simulink model "MaglevOld"  (R2015a)
settings: Solver=ode45  StartTime=0.0  StopTime=10.0  RelTol=1e-3
InitFcn:
  | m = 0.025; % kg
  | g = 9.8; % m/s2
  | L = 0.02; % H
  | R = 4.2; % ohms
  | k = 2.35; % N2/A2
undefined symbols (not defined in the file or in its folder): magnitude
settings Model: Creator=Logan  LastModifiedBy=Logan

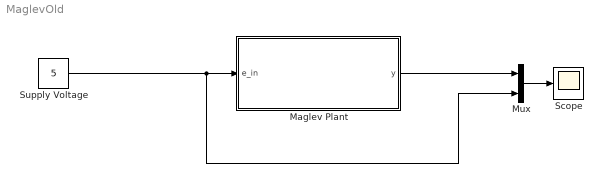
== system MaglevOld ==
  Maglev Plant : Subsystem
  Mux : Mux  Inputs=2
  Scope : Scope
  Supply Voltage : Constant  Value=5
  wires:
  Supply Voltage/1 -> Mux/2, Maglev Plant/1(e_in)
  Maglev Plant/1(y) -> Mux/1
  Mux/1 -> Scope/1

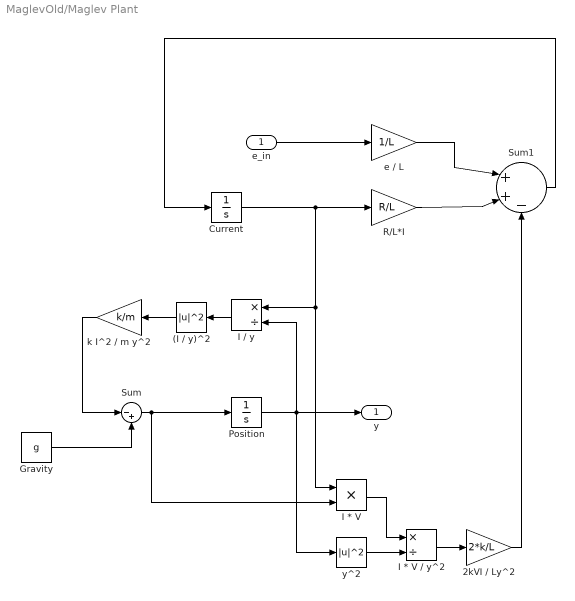
== system MaglevOld/Maglev Plant ==
  e_in : Inport
  (I / y)^2 : Math  Operator=magnitude^2  SaturateOnIntegerOverflow=on
  2kVI / Ly^2 : Gain  Gain=2*k/L
  Current : Integrator  InitialCondition=3.2
  Gravity : Constant  Value=g
  I * V : Product
  I * V / y^2 : Product  Inputs=*/
  I / y : Product  Inputs=*/
  Position : Integrator  InitialCondition=0.01  LimitOutput=on  LowerSaturationLimit=0
  R/L*I : Gain  Gain=R/L
  Sum : Sum  Inputs=|-+
  Sum1 : Sum  Inputs=|++-
  e / L : Gain  Gain=1/L
  k I^2 / m y^2 : Gain  Gain=k/m
  y^2 : Math  Operator=magnitude^2  SaturateOnIntegerOverflow=on
  y : Outport
  wires:
  2kVI / Ly^2/1 -> Sum1/3
  e_in/1 -> e / L/1
  (I / y)^2/1 -> k I^2 / m y^2/1
  e / L/1 -> Sum1/1
  k I^2 / m y^2/1 -> Sum/1
  Sum/1 -> I * V/2, Position/1
  Position/1 -> y^2/1, y/1, I / y/2
  I / y/1 -> (I / y)^2/1
  y^2/1 -> I * V / y^2/2
  Gravity/1 -> Sum/2
  Current/1 -> I / y/1, I * V/1, R/L*I/1
  I * V / y^2/1 -> 2kVI / Ly^2/1
  I * V/1 -> I * V / y^2/1
  R/L*I/1 -> Sum1/2
  Sum1/1 -> Current/1
